simulink model "Non_Linear_Saturated_Control"  (R2024a)
settings: Solver=VariableStepAuto  StartTime=0.0  StopTime=100  RelTol=1e-3
values from neighbouring files (symbols this model uses):
  Gain_Derivative = (2*Damping_Factor*Pulsation_Natural*Time_Constant_Ship - 1)/Static_Gain_Ship    (= -9.85099337748)    [Controller_Rapid_Tuning_Prototype.m]    (also in Robust_PIDF_Tuning_Nichols.m)
  Gain_Filter = 0.01    [Controller_Rapid_Tuning_Prototype.m]    (also in Robust_PIDF_Tuning_Nichols.m)
  Gain_Integral = (Pulsation_Natural^3/2)*(Time_Constant_Ship/Static_Gain_Ship)    (= -0.122930463576)    [Controller_Rapid_Tuning_Prototype.m]    (also in Robust_PIDF_Tuning_Nichols.m)
  Gain_Proportional = (Time_Constant_Ship*Pulsation_Natural^2)/Static_Gain_Ship    (= -0.819536423841)    [Controller_Rapid_Tuning_Prototype.m]    (also in Robust_PIDF_Tuning_Nichols.m)
  Time_Period_Sampling = 0.1    [Controller_Rapid_Tuning_Prototype.m]    (also in Robust_PIDF_Tuning_Nichols.m)
undefined symbols (not defined in the file or in its folder): DiscIntNeverNeededParam
libraries: cstblocks x14
settings Model: Creator=f002706  LastModifiedBy=gerar
settings SolverCC: AlgebraicLoopSolver=TrustRegion
settings DataIOCC: ReturnWorkspaceOutputs=off
settings DebuggingCC: UnconnectedInputMsg=warning  UnconnectedOutputMsg=warning  UnconnectedLineMsg=warning  ArithmeticOperatorsInVariantConditions=warning
settings ModelReferenceCC: EnableRefExpFcnMdlSchedulingChecks=on
settings SFSimCC: SimUseLocalCustomCode=off  CustomCodeUndefinedFunction=UseInterfaceOnly
settings RTWCC: RTWUseLocalCustomCode=off  GPUComputeCapability=3.5
settings CodeAppCC: StateflowObjectComments=on

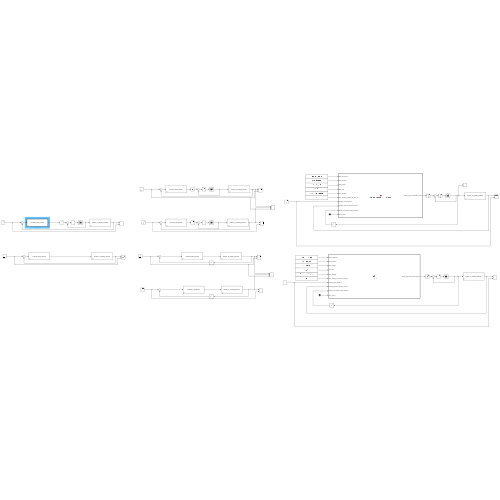
[thumbnail: Simulink's stored preview of the top-level diagram]
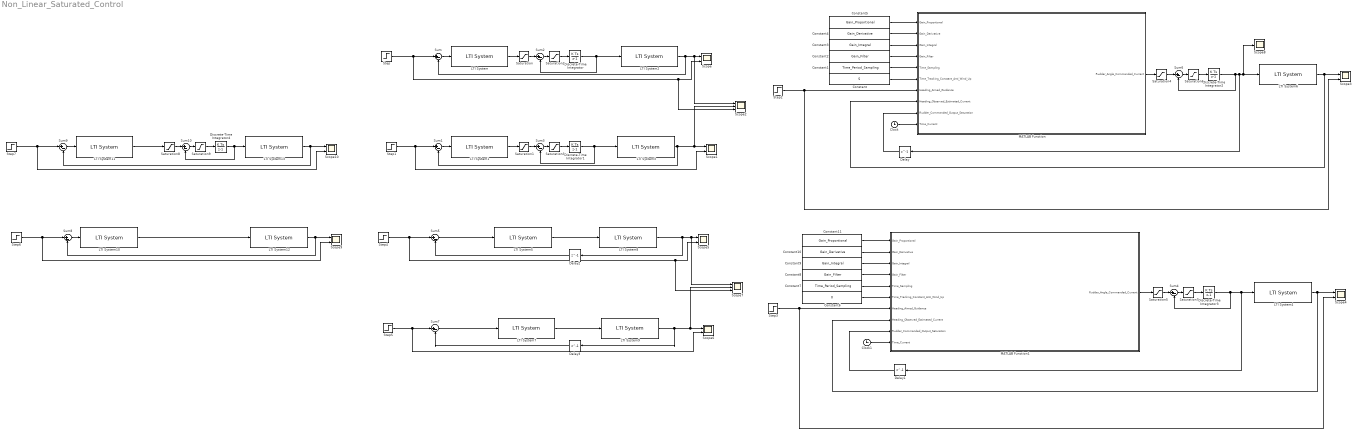
== system Non_Linear_Saturated_Control ==
  Clock : Clock
  Clock1 : Clock
  Constant : Constant  Value=5
  Constant1 : Constant  Value=Time_Period_Sampling
  Constant10 : Constant  Value=Gain_Derivative
  Constant11 : Constant  Value=Gain_Proportional
  Constant2 : Constant  Value=Gain_Filter
  Constant3 : Constant  Value=Gain_Integral
  Constant4 : Constant  Value=Gain_Derivative
  Constant5 : Constant  Value=Gain_Proportional
  Constant6 : Constant  Value=0
  Constant7 : Constant  Value=Time_Period_Sampling
  Constant8 : Constant  Value=Gain_Filter
  Constant9 : Constant  Value=Gain_Integral
  Delay{,1..3} (4 alike) : Delay  DelayLength=1  InputProcessing=Columns as channels (frame based)  SampleTime=Time_Period_Sampling
  Discrete-Time Integrator{,1..4} (5 alike) : DiscreteIntegrator  SampleTime=Time_Period_Sampling  ICPrevOutput=DiscIntNeverNeededParam  ICPrevScaledInput=DiscIntNeverNeededParam
  LTI System : cstblocks/LTI System  sys=Controller_PIDF_Discrete  IC=[]  PadeOrder=0
  LTI System1 : cstblocks/LTI System  sys=Controller_PID_Discrete  IC=[]  PadeOrder=0
  LTI System10 : cstblocks/LTI System  sys=Controller_PDF_Discrete  IC=[]  PadeOrder=0
  LTI System11 : cstblocks/LTI System  sys=Controller_PDF_Discrete  IC=[]  PadeOrder=0
  LTI System{2..4,6,8..9,12..13} (8 alike) : cstblocks/LTI System  sys=Rudder_To_Heading_Discrete  IC=[]  PadeOrder=0
  LTI System5 : cstblocks/LTI System  sys=Controller_PIDF_Discrete  IC=[]  PadeOrder=0
  LTI System7 : cstblocks/LTI System  sys=Controller_PID_Discrete  IC=[]  PadeOrder=0
  MATLAB Function : MATLAB Function  TreatAsAtomicUnit=on  SystemSampleTime=Time_Period_Sampling
  MATLAB Function1 : MATLAB Function  TreatAsAtomicUnit=on  SystemSampleTime=Time_Period_Sampling
  Saturation{,1,4,8} (4 alike) : Saturate  UpperLimit=35*(pi/180)  LowerLimit=-35*(pi/180)
  Saturation2 : Saturate  UpperLimit=20*(pi/180)  LowerLimit=-20*(pi/180)
  Saturation3 : Saturate  UpperLimit=20*(pi/180)  LowerLimit=-20*(pi/180)
  Saturation5 : Saturate  UpperLimit=25*(pi/180)  LowerLimit=-25*(pi/180)
  Saturation6 : Saturate  UpperLimit=5*(pi/180)  LowerLimit=-5*(pi/180)
  Saturation7 : Saturate  UpperLimit=3*(pi/180)  LowerLimit=-3*(pi/180)
  Saturation9 : Saturate  UpperLimit=5*(pi/180)  LowerLimit=-5*(pi/180)
  Scope{,1,3..6,9..10} (8 alike) : Scope  NumInputPorts=2
  Scope2 : Scope  NumInputPorts=3
  Scope7 : Scope  NumInputPorts=3
  Scope8 : Scope
  Step{,1..7} (8 alike) : Step  After=25*(pi/180)  SampleTime=0
  Sum{,1..10} (11 alike) : Sum  Inputs=|+-
  wires:
  LTI System1/1 -> Saturation1/1
  LTI System/1 -> Saturation/1
  LTI System2/1 -> Scope2/1, Scope/1, Sum/2
  LTI System3/1 -> Sum1/2, Scope2/2, Scope1/1
  Sum/1 -> LTI System/1
  Sum1/1 -> LTI System1/1
  Step/1 -> Scope2/3, Scope/2, Sum/1
  Step1/1 -> Scope1/2, Sum1/1
  Saturation2/1 -> Discrete-Time Integrator/1
  Saturation3/1 -> Discrete-Time Integrator1/1
  Discrete-Time Integrator/1 -> Sum2/2, LTI System2/1
  Discrete-Time Integrator1/1 -> Sum3/2, LTI System3/1
  Saturation/1 -> Sum2/1
  Sum2/1 -> Saturation2/1
  Saturation1/1 -> Sum3/1
  Sum3/1 -> Saturation3/1
  Step2/1 -> MATLAB Function/7(Heading_Aimed_Guidance), Scope3/2
  Saturation4/1 -> Sum6/1
  Saturation6/1 -> Discrete-Time Integrator2/1
  LTI System6/1 -> MATLAB Function/8(Heading_Observed_Estimated_Current), Scope3/1
  Sum6/1 -> Saturation6/1
  MATLAB Function/1(Rudder_Angle_Commanded_Current) -> Saturation4/1
  Discrete-Time Integrator2/1 -> Sum6/2, Delay/1, Scope8/1, LTI System6/1
  Clock/1 -> MATLAB Function/10(Time_Current)
  Delay/1 -> MATLAB Function/9(Rudder_Commanded_Output_Saturation)
  Constant/1 -> MATLAB Function/6(Time_Tracking_Constant_Anti_Wind_Up)
  Constant1/1 -> MATLAB Function/5(Time_Sampling)
  Constant2/1 -> MATLAB Function/4(Gain_Filter)
  Constant3/1 -> MATLAB Function/3(Gain_Integral)
  Constant4/1 -> MATLAB Function/2(Gain_Derivative)
  Constant5/1 -> MATLAB Function/1(Gain_Proportional)
  Constant6/1 -> MATLAB Function1/6(Time_Tracking_Constant_Anti_Wind_Up)
  Clock1/1 -> MATLAB Function1/10(Time_Current)
  MATLAB Function1/1(Rudder_Angle_Commanded_Current) -> Saturation5/1
  LTI System4/1 -> MATLAB Function1/8(Heading_Observed_Estimated_Current), Scope4/1
  Saturation7/1 -> Discrete-Time Integrator3/1
  Saturation5/1 -> Sum4/1
  Discrete-Time Integrator3/1 -> Sum4/2, Delay1/1, LTI System4/1
  Step3/1 -> MATLAB Function1/7(Heading_Aimed_Guidance), Scope4/2
  Sum4/1 -> Saturation7/1
  Delay1/1 -> MATLAB Function1/9(Rudder_Commanded_Output_Saturation)
  Constant7/1 -> MATLAB Function1/5(Time_Sampling)
  Constant8/1 -> MATLAB Function1/4(Gain_Filter)
  Constant9/1 -> MATLAB Function1/3(Gain_Integral)
  Constant10/1 -> MATLAB Function1/2(Gain_Derivative)
  Constant11/1 -> MATLAB Function1/1(Gain_Proportional)
  Step4/1 -> Scope7/3, Scope5/2, Sum5/1
  Step5/1 -> Scope6/2, Sum7/1
  Sum7/1 -> LTI System7/1
  Sum5/1 -> LTI System5/1
  LTI System9/1 -> Delay3/1, Scope7/2, Scope6/1
  LTI System8/1 -> Scope7/1, Scope5/1, Delay2/1
  LTI System5/1 -> LTI System8/1
  LTI System7/1 -> LTI System9/1
  LTI System10/1 -> LTI System12/1
  Step6/1 -> Scope9/2, Sum8/1
  LTI System12/1 -> Scope9/1, Sum8/2
  Sum8/1 -> LTI System10/1
  Sum9/1 -> LTI System11/1
  Step7/1 -> Scope10/2, Sum9/1
  LTI System13/1 -> Scope10/1, Sum9/2
  Saturation8/1 -> Sum10/1
  Saturation9/1 -> Discrete-Time Integrator4/1
  Sum10/1 -> Saturation9/1
  LTI System11/1 -> Saturation8/1
  Discrete-Time Integrator4/1 -> Sum10/2, LTI System13/1
  Delay2/1 -> Sum5/2
  Delay3/1 -> Sum7/2

== matlab function Non_Linear_Saturated_Control/MATLAB Function1 ==
  data: Gain_Proportional input; Rudder_Angle_Commanded_Current output; Gain_Derivative input; Gain_Integral input; Gain_Filter input; Time_Sampling input; Time_Tracking_Constant_Anti_Wind_Up input; Heading_Aimed_Guidance input; Heading_Observed_Estimated_Current input; Rudder_Commanded_Output_Saturation input; Time_Current input
function Rudder_Angle_Commanded_Current  = PIDF_Anti_Wind_Up_Incremental(Gain_Proportional,...
                   Gain_Derivative,...
                   Gain_Integral,...
                   Gain_Filter,...
                   Time_Sampling,...
                   Time_Tracking_Constant_Anti_Wind_Up,...
                   Heading_Aimed_Guidance,...
                   Heading_Observed_Estimated_Current,...
                   Rudder_Commanded_Output_Saturation,...
                   Time_Current)

% Persistents definition:
persistent Control_Increment_Previous;
persistent Heading_Error_Previous;
persistent Heading_Error_Previous_Previous;
persistent Count_Iteration;
persistent Control_Signal_Previous;

% Persistents initialization:
if isempty(Control_Increment_Previous)
	Control_Increment_Previous = 0;
end
if isempty(Heading_Error_Previous)
	Heading_Error_Previous = 0;
end
if isempty(Heading_Error_Previous_Previous)
	Heading_Error_Previous_Previous = 0;
end
if isempty(Count_Iteration)
	Count_Iteration = 0;
end
if isempty(Control_Signal_Previous)
	Control_Signal_Previous = 0;
end

% Hardcoded limits:
Rudder_Angle_Maximal_Saturated = 25*(pi/180);
Rudder_Angle_Minimal_Saturated = -25*(pi/180);

% Controller gains declaration:
Controller_Zero_Gain_0 = (Gain_Proportional*(Time_Sampling + Gain_Filter) + Gain_Integral*(Time_Sampling^2 + Time_Sampling*Gain_Filter) + ...
						  Gain_Derivative)/(Time_Sampling + Gain_Filter);
						  
Controller_Zero_Gain_1 = (Gain_Proportional*(-2*Gain_Filter - Time_Sampling) - Gain_Integral*Time_Sampling*Gain_Filter - 2*Gain_Derivative)/...
					     (Time_Sampling + Gain_Filter);
						 
Controller_Zero_Gain_2 = (Gain_Proportional*Gain_Filter + Gain_Derivative)/(Time_Sampling + Gain_Filter);

Controller_Pole_Gain_Beta = Gain_Filter/(Time_Sampling + Gain_Filter);

% Calculation of the current heading error:
Heading_Error_Current = Heading_Aimed_Guidance - Heading_Observed_Estimated_Current;

% Calculate the control increment:
Control_Increment_Current = Controller_Pole_Gain_Beta*Control_Increment_Previous + Controller_Zero_Gain_0*Heading_Error_Current + ...
							Controller_Zero_Gain_1*Heading_Error_Previous + Controller_Zero_Gain_2*Heading_Error_Previous_Previous;
							
% Then calculate the control signal:
Control_Signal_Current = Control_Increment_Current + Control_Signal_Previous;

% Safe definition of the output of the saturation at the first time step:
if Time_Current == 0
	Rudder_Commanded_Output_Saturation = 0;
end

% Conditional output update:
if Control_Signal_Current > Rudder_Angle_Maximal_Saturated || ...
	Control_Signal_Current < Rudder_Angle_Minimal_Saturated
	Control_Increment_Current = Rudder_Commanded_Output_Saturation - Control_Signal_Previous;
	% Output:
	Rudder_Angle_Commanded_Current = Rudder_Commanded_Output_Saturation;
else
	Rudder_Angle_Commanded_Current = Control_Signal_Current;
end

% Persistents update:																			
Control_Increment_Previous = Control_Increment_Current;
Count_Iteration = Count_Iteration + 1;
if Count_Iteration == 1
    Heading_Error_Previous_Previous = 0;
else
    Heading_Error_Previous_Previous = Heading_Error_Previous;
end
Heading_Error_Previous = Heading_Error_Current;	
Control_Signal_Previous = Rudder_Angle_Commanded_Current;	

end

== matlab function Non_Linear_Saturated_Control/MATLAB Function ==
  data: Gain_Proportional input; Rudder_Angle_Commanded_Current output; Gain_Derivative input; Gain_Integral input; Gain_Filter input; Time_Sampling input; Time_Tracking_Constant_Anti_Wind_Up input; Heading_Aimed_Guidance input; Heading_Observed_Estimated_Current input; Rudder_Commanded_Output_Saturation input; Time_Current input
function Rudder_Angle_Commanded_Current  = PIDF_Anti_Wind_Up_Back_Calculation(Gain_Proportional,...
                      Gain_Derivative,...
                      Gain_Integral,...
                      Gain_Filter,...
                      Time_Sampling,...
                      Time_Tracking_Constant_Anti_Wind_Up,...
                      Heading_Aimed_Guidance,...
                      Heading_Observed_Estimated_Current,...
                      Rudder_Commanded_Output_Saturation,...
                      Time_Current)

% Persistents definition:
persistent Input_Command_Integral_Previous;
persistent Input_Command_Derivative_Previous;
persistent Heading_Error_Previous

% Persistents initialization:
if isempty(Input_Command_Integral_Previous)
	Input_Command_Integral_Previous = 0;
end
if isempty(Input_Command_Derivative_Previous)
	Input_Command_Derivative_Previous = 0;
end
if isempty(Heading_Error_Previous)
	Heading_Error_Previous = 0;
end

% Calculation of the current heading error:
Heading_Error_Current = Heading_Aimed_Guidance - Heading_Observed_Estimated_Current;

% Update the commanded inputs for each actions:
% Proportional:
Input_Command_Proportional_Current = Gain_Proportional*Heading_Error_Current;

% Integral:
Input_Command_Integral_Current = Input_Command_Integral_Previous + Gain_Integral*Time_Sampling*Heading_Error_Current;

% Derivative:
Input_Command_Derivative_Current = (Gain_Derivative*(Heading_Error_Current - Heading_Error_Previous) + ...
									Gain_Filter*Input_Command_Derivative_Previous)/(Gain_Filter + Time_Sampling);
									
% Establish the current control signal:
Control_Input_Signal_No_Wind_Up = Input_Command_Proportional_Current + Input_Command_Integral_Current + Input_Command_Derivative_Current;

% Current error between output of saturation and output of the controller:
if Time_Current == 0
	% Then first time step point:
	Rudder_Commanded_Output_Saturation = 0; % Protection for the first time step.
end
Error_Anti_Wind_Up_Current = Rudder_Commanded_Output_Saturation - Control_Input_Signal_No_Wind_Up;

% Back-calculation integral term anti wind-up protection:
Input_Command_Integral_Anti_Wind_Up_Current = Input_Command_Integral_Previous + (Gain_Integral*Heading_Error_Current + ...
										      (1/Time_Tracking_Constant_Anti_Wind_Up)*Error_Anti_Wind_Up_Current)*Time_Sampling;
											  
% Then calculate the new input signal if the saturation is activated: 
Control_Input_Signal_Wind_Up = Input_Command_Proportional_Current + Input_Command_Integral_Anti_Wind_Up_Current + Input_Command_Derivative_Current;

% Output of the algorithm:
Rudder_Angle_Commanded_Current = Control_Input_Signal_Wind_Up;

% Persistents update:
Input_Command_Integral_Previous = Input_Command_Integral_Anti_Wind_Up_Current; % But also try Input_Command_Integral_Current.
Input_Command_Derivative_Previous = Input_Command_Derivative_Current;
Heading_Error_Previous = Heading_Error_Current;

end
